simulink model "remoteFly_v1"  (R2018b)
settings: Solver=FixedStepAuto  StartTime=0.0  StopTime=inf  RelTol=1e-3  EnableMultiTasking=on
undefined symbols (not defined in the file or in its folder): ch1_thrust, ch2_Ail, ch3_Ele, ch4_SC, ch5_S1, ch6_S2, ch7_LS, ch8_RS, dev, Main, pwm_output0
libraries: simulink x2, px4Sensorslib x2, px4lib x1, sharedtransform x1
settings Model: SimulationMode=external  ExtModeTrigDuration=10  Creator=Robert  LastModifiedBy=Robert
settings SolverCC: PositivePriorityOrder=on
settings OptimizationCC: EnhancedBackFolding=on  PassReuseOutputArgsAs=Individual arguments  MaxStackSize=64  OptimizeBlockOrder=speed  DifferentSizesBufferReuse=on  OptimizationCustomize=off
settings DebuggingCC: ParameterTunabilityLossMsg=error
settings HardwareCC: ProdBitPerPointer=32  ProdBitPerSizeT=32  ProdBitPerPtrDiffT=32  ProdLargestAtomicInteger=Long  ProdLargestAtomicFloat=Double  ProdWordSize=32  ProdLongLongMode=on  ProdHWDeviceType=ARM Compatible->ARM Cortex
settings SFSimCC: MATLABDynamicMemAlloc=off
settings RTWCC: SystemTargetFile=ert.tlc  HardwareBoard=PX4 Pixhawk 1  TLCOptions="-aInlineSetEventsForThisBaseRateFcn=TLC_FALSE -aSuppressMultiTaskScheduler=TLC_FALSE  -aRateBasedStepFcn=0"  TemplateMakefile=ert_default_tmf  GenerateReport=on  Toolchain=GNU Tools for PX4 Autopilots  IncludeHyperlinkInReport=on  LaunchReport=on  TargetLang=C++  GenerateTraceInfo=on  GenerateTraceReport=on  GenerateTraceReportSl=on  GenerateTraceReportSf=on  GenerateTraceReportEml=on
settings CodeAppCC: ForceParamTrailComments=on  IgnoreCustomStorageClasses=off  OperatorAnnotations=on  SimulinkDataObjDesc=on  SFDataObjDesc=on  InsertBlockDesc=on
settings ERTTargetCC: ExtMode=on  ExtModeMexArgs='127.0.0.1' 1 17725

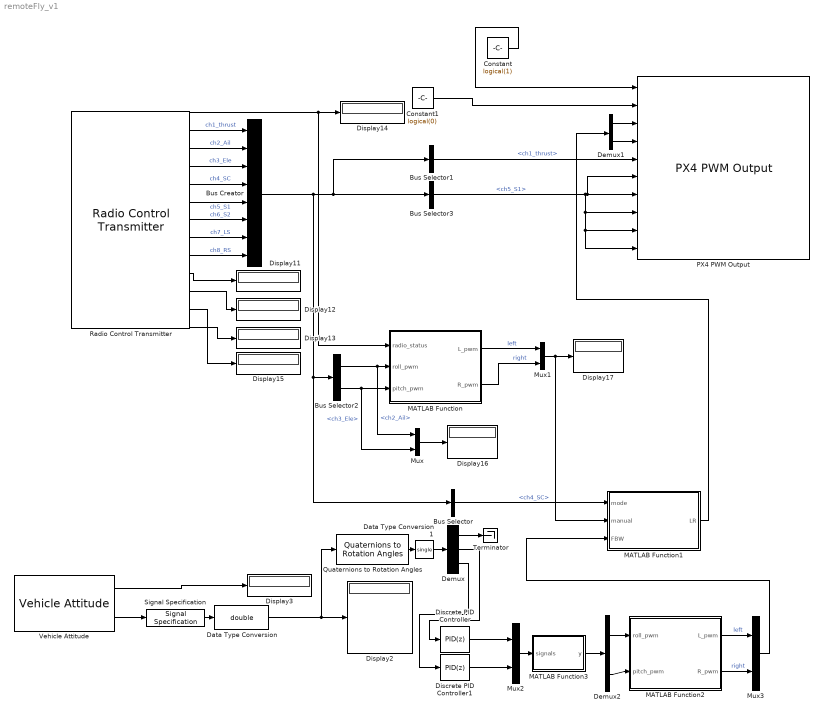
== system remoteFly_v1 ==
  Bus Creator : BusCreator  Inputs=ch1_thrust,ch2_Ail,ch3_Ele,ch4_SC,ch5_S1,ch6_S2,ch7_LS,ch8_RS
  Bus Selector : BusSelector  OutputSignals=ch4_SC
  Bus Selector1 : BusSelector  OutputSignals=ch1_thrust
  Bus Selector2 : BusSelector  OutputSignals=ch2_Ail,ch3_Ele
  Bus Selector3 : BusSelector  OutputSignals=ch5_S1
  Constant : Constant  Value=logical(1)
  Constant1 : Constant  Value=logical(0)
  Data Type Conversion : DataTypeConversion  OutDataTypeStr=double
  Data Type Conversion1 : DataTypeConversion  OutDataTypeStr=single
  Demux : Demux  Outputs=3
  Demux1 : Demux  Outputs=2
  Demux2 : Demux  Outputs=2
  Discrete PID Controller : simulink/Continuous/PID Controller  Controller=PID  Form=Parallel  TimeDomain=Discrete-time  SampleTime=-1  IntegratorMethod=Forward Euler  FilterMethod=Forward Euler  ControllerParametersSource=internal  P=1  I=0  D=0  UseFilter=on  N=100  TunerSelectOption=Transfer Function Based (PID Tuner App)  InitialConditionSource=internal  InitialConditionForIntegrator=0  InitialConditionForFilter=0  DifferentiatorICPrevScaledInput=0  ExternalReset=none  TrackingMode=off  Kt=1  LimitOutput=on  UpperSaturationLimit=1  LowerSaturationLimit=-1  LinearizeAsGain=off  AntiWindupMode=none  Kb=1  POutMin=[]  POutMax=[]  IOutMin=[]  IOutMax=[]  DOutMin=[]  DOutMax=[]  NOutMin=[]  NOutMax=[]  SumOutMin=[]  SumOutMax=[]  SaturationOutMin=[]  SaturationOutMax=[]  PParamMin=[]  PParamMax=[]  IParamMin=[]  IParamMax=[]  DParamMin=[]  DParamMax=[]  NParamMin=[]  NParamMax=[]  KbParamMin=[]  KbParamMax=[]  KtParamMin=[]  KtParamMax=[]  KbOutMin=[]  KbOutMax=[]  KtOutMin=[]  KtOutMax=[]  IntegratorOutMin=[]  IntegratorOutMax=[]  FilterOutMin=[]  FilterOutMax=[]  SumI1OutMin=[]  SumI1OutMax=[]  SumI2OutMin=[]  SumI2OutMax=[]  SumI3OutMin=[]  SumI3OutMax=[]  SumI4OutMin=[]  SumI4OutMax=[]  SumDOutMin=[]  SumDOutMax=[]  DifferentiatorOutMin=[]  DifferentiatorOutMax=[]  FilterDiffOutCoefMin=[]  FilterDiffOutCoefMax=[]  ReciprocalOutMin=[]  ReciprocalOutMax=[]  SumDenOutMin=[]  SumDenOutMax=[]  SumNumOutMin=[]  SumNumOutMax=[]  DivideOutMin=[]  DivideOutMax=[]  IntegratorContinuousStateAttributes=''  IntegratorStateMustResolveToSignalObject=off  IntegratorRTWStateStorageClass=Auto  FilterContinuousStateAttributes=''  FilterStateMustResolveToSignalObject=off  FilterRTWStateStorageClass=Auto  ParallelPVariant=InternalParameters  IdealPVariant=Disabled  IVariant=InternalParameters  DVariant=InternalParameters  IntegratorVariant=Discrete  SatVariant=Enabled  AWVariant=Passthrough  PCopyVariant=Disabled  TRVariant=Disabled  FdbkBlocksVariant=Forward  IdealPFdbkVariant=Disabled  SatFdbkVariant=Disabled  DerivativeFilterVariant=ForwardEulerFilter  NVariant=InternalParameters  NCopyVariant=Disabled  FilterICVariant=InternalICsFilter  IntegratorICVariant=InternalICs  ExternalResetVariant=Disabled  TRSumVariant=Passthrough  SumFdbkVariant=Disabled  SumVariant=Sum_PID
  Discrete PID Controller1 : simulink/Continuous/PID Controller  Controller=PID  Form=Parallel  TimeDomain=Discrete-time  SampleTime=-1  IntegratorMethod=Forward Euler  FilterMethod=Forward Euler  ControllerParametersSource=internal  P=1  I=0  D=0  UseFilter=on  N=100  TunerSelectOption=Transfer Function Based (PID Tuner App)  InitialConditionSource=internal  InitialConditionForIntegrator=0  InitialConditionForFilter=0  DifferentiatorICPrevScaledInput=0  ExternalReset=none  TrackingMode=off  Kt=1  LimitOutput=on  UpperSaturationLimit=1  LowerSaturationLimit=-1  LinearizeAsGain=off  AntiWindupMode=none  Kb=1  POutMin=[]  POutMax=[]  IOutMin=[]  IOutMax=[]  DOutMin=[]  DOutMax=[]  NOutMin=[]  NOutMax=[]  SumOutMin=[]  SumOutMax=[]  SaturationOutMin=[]  SaturationOutMax=[]  PParamMin=[]  PParamMax=[]  IParamMin=[]  IParamMax=[]  DParamMin=[]  DParamMax=[]  NParamMin=[]  NParamMax=[]  KbParamMin=[]  KbParamMax=[]  KtParamMin=[]  KtParamMax=[]  KbOutMin=[]  KbOutMax=[]  KtOutMin=[]  KtOutMax=[]  IntegratorOutMin=[]  IntegratorOutMax=[]  FilterOutMin=[]  FilterOutMax=[]  SumI1OutMin=[]  SumI1OutMax=[]  SumI2OutMin=[]  SumI2OutMax=[]  SumI3OutMin=[]  SumI3OutMax=[]  SumI4OutMin=[]  SumI4OutMax=[]  SumDOutMin=[]  SumDOutMax=[]  DifferentiatorOutMin=[]  DifferentiatorOutMax=[]  FilterDiffOutCoefMin=[]  FilterDiffOutCoefMax=[]  ReciprocalOutMin=[]  ReciprocalOutMax=[]  SumDenOutMin=[]  SumDenOutMax=[]  SumNumOutMin=[]  SumNumOutMax=[]  DivideOutMin=[]  DivideOutMax=[]  IntegratorContinuousStateAttributes=''  IntegratorStateMustResolveToSignalObject=off  IntegratorRTWStateStorageClass=Auto  FilterContinuousStateAttributes=''  FilterStateMustResolveToSignalObject=off  FilterRTWStateStorageClass=Auto  ParallelPVariant=InternalParameters  IdealPVariant=Disabled  IVariant=InternalParameters  DVariant=InternalParameters  IntegratorVariant=Discrete  SatVariant=Enabled  AWVariant=Passthrough  PCopyVariant=Disabled  TRVariant=Disabled  FdbkBlocksVariant=Forward  IdealPFdbkVariant=Disabled  SatFdbkVariant=Disabled  DerivativeFilterVariant=ForwardEulerFilter  NVariant=InternalParameters  NCopyVariant=Disabled  FilterICVariant=InternalICsFilter  IntegratorICVariant=InternalICs  ExternalResetVariant=Disabled  TRSumVariant=Passthrough  SumFdbkVariant=Disabled  SumVariant=Sum_PID
  Display{2..3,11..17} (9 alike) : Display
  MATLAB Function : MATLAB Function  TreatAsAtomicUnit=on
  MATLAB Function1 : MATLAB Function  TreatAsAtomicUnit=on
  MATLAB Function2 : MATLAB Function  TreatAsAtomicUnit=on
  MATLAB Function3 : MATLAB Function  TreatAsAtomicUnit=on
  Mux{,1..3} (4 alike) : Mux  Inputs=2
  PX4 PWM Output : px4lib/PX4 PWM Output  pwmDevice=Main (/dev/pwm_output0)  pwmChannel1_=on  pwmChannel2_=on  pwmChannel3_=on  pwmChannel4_=on  pwmChannel5_=on  pwmChannel6_=on  pwmChannel7_=on  pwmChannel8_=on  forceTerminateFailsafe=off  outputErrorStatus=off
      settings: SourceProductName=Embedded Coder Support Package for PX4 Autopilots
  Quaternions to Rotation Angles : sharedtransform/Quaternions to Rotation Angles  rotationOrder=ZYX  aMode=aMode
      settings: SourceProductBaseCode=AE
  Radio Control Transmitter : px4Sensorslib/Radio Control Transmitter  channel1=on  channel2=on  channel3=on  channel4=on  channel5=on  channel6=on  channel7=on  channel8=on  channel_count=on  rssi=on  rc_input_source=on  timestamp_last_signal=on  time_stamp=off  sampleTime=1/250  BlockingMode=off  BlockTimeout=5
      settings: SourceProductName=Embedded Coder Support Package for PX4 Autopilots
  Signal Specification : SignalSpecification  OutDataTypeStr=single
  Terminator : Terminator
  Vehicle Attitude : px4Sensorslib/Vehicle Attitude  rollRate=off  pitchRate=off  yawRate=off  quaternion=on  uorbTimeStamp=off  BlockingMode=off  BlockTimeout=0.001  sampleTime=1/250
      settings: SourceProductName=Embedded Coder Support Package for PX4 Autopilots
  wires:
  Vehicle Attitude/2 -> Signal Specification/1
  Vehicle Attitude/1 -> Display3/1
  Radio Control Transmitter/8 -> Bus Creator/7  "ch7_LS"
  Radio Control Transmitter/7 -> Bus Creator/6  "ch6_S2"
  Radio Control Transmitter/6 -> Bus Creator/5  "ch5_S1"
  Radio Control Transmitter/2 -> Bus Creator/1  "ch1_thrust"
  Radio Control Transmitter/3 -> Bus Creator/2  "ch2_Ail"
  Radio Control Transmitter/4 -> Bus Creator/3  "ch3_Ele"
  Radio Control Transmitter/5 -> Bus Creator/4  "ch4_SC"
  Radio Control Transmitter/9 -> Bus Creator/8  "ch8_RS"
  Radio Control Transmitter/10 -> Display11/1
  Radio Control Transmitter/11 -> Display12/1
  Radio Control Transmitter/13 -> Display13/1
  Radio Control Transmitter/1 -> MATLAB Function/1(radio_status), Display14/1
  Radio Control Transmitter/12 -> Display15/1
  Constant/1 -> PX4 PWM Output/1
  MATLAB Function/1(L_pwm) -> Mux1/1  "left"
  MATLAB Function/2(R_pwm) -> Mux1/2  "right"
  Bus Selector1/1 -> PX4 PWM Output/5  "<ch1_thrust>"
  Bus Selector3/1 -> PX4 PWM Output/10, PX4 PWM Output/9, PX4 PWM Output/8, PX4 PWM Output/7, PX4 PWM Output/6  "<ch5_S1>"
  Constant1/1 -> PX4 PWM Output/2
  Bus Creator/1 -> Bus Selector3/1, Bus Selector1/1, Bus Selector/1, Bus Selector2/1
  Bus Selector2/1 -> MATLAB Function/2(roll_pwm), Mux/1  "<ch2_Ail>"
  Bus Selector2/2 -> MATLAB Function/3(pitch_pwm), Mux/2  "<ch3_Ele>"
  Mux/1 -> Display16/1
  Mux1/1 -> MATLAB Function1/2(manual), Display17/1
  Quaternions to Rotation Angles/1 -> Data Type Conversion1/1
  Demux/1 -> Terminator/1
  Demux1/1 -> PX4 PWM Output/3
  Demux1/2 -> PX4 PWM Output/4
  MATLAB Function1/1(LR) -> Demux1/1
  Bus Selector/1 -> MATLAB Function1/1(mode)  "<ch4_SC>"
  Demux/2 -> Discrete PID Controller/1
  Demux/3 -> Discrete PID Controller1/1
  Discrete PID Controller1/1 -> Mux2/2
  Discrete PID Controller/1 -> Mux2/1
  Mux2/1 -> MATLAB Function3/1(signals)
  Demux2/2 -> MATLAB Function2/2(pitch_pwm)
  Demux2/1 -> MATLAB Function2/1(roll_pwm)
  MATLAB Function3/1(y) -> Demux2/1
  MATLAB Function2/1(L_pwm) -> Mux3/1  "left"
  MATLAB Function2/2(R_pwm) -> Mux3/2  "right"
  Mux3/1 -> MATLAB Function1/3(FBW)
  Data Type Conversion/1 -> Quaternions to Rotation Angles/1, Display2/1
  Signal Specification/1 -> Data Type Conversion/1
  Data Type Conversion1/1 -> Demux/1

== matlab function remoteFly_v1/MATLAB Function1 ==
  data: mode input; LR output uint16; manual input; FBW input
function LR = fcn(mode, manual, FBW)

if mode<1400
    LR = manual;
elseif mode<1600
    LR = FBW;
else
    LR = uint16([1500,1500]');
end

== matlab function remoteFly_v1/MATLAB Function ==
  data: radio_status input; roll_pwm input; L_pwm output; pitch_pwm input; R_pwm output
function [L_pwm,R_pwm] = pitch_roll_pwmTranslator(radio_status, roll_pwm,pitch_pwm)
%{
First subtract center point for PWM
Then remember servos are mounted in different orientations.
On right wing positive -> elevon down.
On left wing positive -> elevon up
Finally add back center point

Pitch up -> PWM negative -> correct sign for right, invert for left.
Roll right -> PWM positive -> invert for left, invert for right
%}

% Radio status:
% 0=new message
% 1=holding last message
% 2=rc_failsafe
% 3= 1 and 2.
% 4=rc_lost

neutral = single(1500);
% At startup the radio may indicate holding last value,
% which in memory will be 0 and thus not viable.
if (radio_status==0 || radio_status==1) && roll_pwm~=0 && pitch_pwm~=0

    roll    =  single(roll_pwm)  - neutral;
    pitch   =  single(pitch_pwm) - neutral;
    L       = -pitch - roll + neutral;
    R       =  pitch - roll + neutral;
    L_pwm       = uint16(L);
    R_pwm       = uint16(R);
else
    L_pwm       = uint16(neutral);
    R_pwm       = uint16(neutral);
end

%L_pwm = -pitch_pwm -roll_pwm + 3*neutral;
%R_pwm = pitch_pwm  - roll_pwm + neutral; % The neutrals cancel

end

== matlab function remoteFly_v1/MATLAB Function2 ==
  data: roll_pwm input; L_pwm output; pitch_pwm input; R_pwm output
function [L_pwm,R_pwm] = pitch_roll_pwmTranslator(roll_pwm,pitch_pwm)
%{
First subtract center point for PWM
Then remember servos are mounted in different orientations.
On right wing positive -> elevon down.
On left wing positive -> elevon up
Finally add back center point

Pitch up -> PWM negative -> correct sign for right, invert for left.
Roll right -> PWM positive -> invert for left, invert for right
%}

% Radio status:
% 0=new message
% 1=holding last message
% 2=rc_failsafe
% 3= 1 and 2.
% 4=rc_lost

neutral = single(1500);
% At startup the radio may indicate holding last value,
% which in memory will be 0 and thus not viable.

roll    =  single(roll_pwm)  - neutral;
pitch   =  single(pitch_pwm) - neutral;
L       = -pitch - roll + neutral;
R       =  pitch - roll + neutral;
L_pwm       = uint16(L);
R_pwm       = uint16(R);


%L_pwm = -pitch_pwm -roll_pwm + 3*neutral;
%R_pwm = pitch_pwm  - roll_pwm + neutral; % The neutrals cancel

end

== matlab function remoteFly_v1/MATLAB Function3 ==
  data: signals input; y output
function y = signal2pwm(signals)

y = uint16(zeros(size(signals)));


% Range is ~1000-2000, ie +-500, but in is +-1
signals = signals.*500;
% Shift to center PWM
signals = signals+1500;
y = uint16(signals);
